simulink library "tqd"  (R2021b)
settings: Solver=VariableStepAuto  StartTime=0.0  StopTime=10.0  RelTol=1e-3
undefined symbols (not defined in the file or in its folder): ATQD_AccelLimitInRange_X_rpm, ATQD_AccelLimitInRange_Y_Nm, ATQD_AccelLimitOvrKi_X_Nm, ATQD_AccelLimitOvrKp_X_Nm, ATQD_BOSMapD_X_rpm, ATQD_BOSMapD_Y_pct, ATQD_BOSMapR_X_rpm, ATQD_BOSMapR_Y_pct, ATQD_HVBCurrSmooth_X_A, ATQD_LHMTqMapDLC_X_rpm, ATQD_LHMTqMapDLC_Y_pct, ATQD_LHMTqMapRLC_X_rpm, ATQD_LHMTqMapRLC_Y_pct, ATQD_NormalMapDLC_X_rpm, ATQD_NormalMapDLC_Y_pct, ATQD_NormalTqDecSR_X_rpm, ATQD_NormalTqDecSR_Y_Nm, ATQD_NormalTqIncSR_X_rpm, ATQD_NormalTqIncSR_Y_Nm, ATQD_OPDMapRLC_X_rpm, ATQD_OPDMapRLC_Y_pct, ATQD_RollRegTorReq_X_rpm, ATQD_RollRegTorReq_Y_enum, ATQD_VehSpdLimitInRange_X_rpm, ATQD_VehSpdLimitInRange_Y_Nm, ATQD_VehSpdLimitOvrKi_X_Nm, ATQD_VehSpdLimitOvrKp_X_Nm, EIGHT_INT, ENUM_BRAKEPEDAL_PRESSED, ENUM_BRAKEPEDAL_RELEASED, ENUM_COMBOKEY_DOWN, ENUM_COMBOKEY_M1, ENUM_COMBOKEY_M2, ENUM_COMBOKEY_NONE, ENUM_COMBOKEY_RKNEE, ENUM_COMBOKEY_STOPLV, ENUM_COMBOKEY_UP, ENUM_CP2VKNEEREQ_REQUEST, ENUM_CP2VNLVREQ_LEVEL1, ENUM_CP2VNLVREQ_LEVEL2, ENUM_CP2VNLVREQ_LOWER, ENUM_CP2VNLVREQ_STOPLV, ENUM_CP2VNLVREQ_UPPER, ENUM_CREEPIND_DISABLE, ENUM_CREEPIND_READY, ENUM_CREEPIND_RUNNING, ENUM_CREEPIND_WARNING, ENUM_DRIVELINERELEASE_RELEASE, ENUM_EBSTORQUERWQ_LIMIT, ENUM_EBSTORQUERWQ_TORQUE, ENUM_ECPVCUDRM_CONFORT, ENUM_ECPVCUDRM_ECO, ENUM_ECPVCUDRM_NORMAL, ENUM_ECPVCUDRM_NOTAVAILABLE, ENUM_EMTqModeDrvBrk_Accel, ENUM_EMTqModeDrvBrk_Brake, ENUM_EMTqModeDrvBrk_Coast, ENUM_ETC2ACTDRIVEDIR_BACKWARD, ENUM_ETC2ACTDRIVEDIR_FORWARD, ENUM_ETC2ACTDRIVEDIR_STILL ... (+341)
libraries: simulink x109, hcu_lib x67
(part 8 of 13)

== system tqd/TQD/OutpConvert/Buzzer Request/Parking Protect Flasher ==
  Task_Time_s : Inport
  ON_s : Inport  Port=2
  OFF_s : Inport  Port=3
  Cycle_cnt : Inport  Port=4
  Wait_s : Inport  Port=5
  VSCP_FlasherEn_flg : Inport  Port=6
  Add : Sum  Inputs=+-
  Chart : Stateflow chart  TreatAsAtomicUnit=on
  Constant4 : Constant  Value=ONE_INT
  Data Type Conversion{,1..3} (4 alike) : DataTypeConversion  OutDataTypeStr=uint8
  Divide : Product  Inputs=*/
  Divide1 : Product  Inputs=*/
  Divide2 : Product  Inputs=*/
  Floor : Rounding
  Floor1 : Rounding
  Floor2 : Rounding
  SigOut : Outport
  wires:
  Floor/1 -> Data Type Conversion/1  "ON_cnt"
  [TaskTime_s] -> Divide2/2
  [Cycle_cnt] -> Add/1  "Cycle_cnt"
  VSCP_FlasherEn_flg/1 -> [VSCP_FlasherEn_flg]
  [VSCP_FlasherEn_flg] -> Chart/5(VSCP_FlasherEn_flg)
  Wait_s/1 -> [Wait_s]
  Task_Time_s/1 -> [TaskTime_s]
  OFF_s/1 -> [OFF_s]
  Cycle_cnt/1 -> [Cycle_cnt]
  [TaskTime_s] -> Divide/2
  [Wait_s] -> Divide2/1  "Wait_s"
  [OFF_s] -> Divide1/1  "OFF_s"
  Constant4/1 -> Add/2
  Data Type Conversion3/1 -> Chart/4(Cycle_cnt)
  ON_s/1 -> [ON_s]
  Divide1/1 -> Floor1/1
  Floor2/1 -> Data Type Conversion2/1  "WAIT_cnt"
  [ON_s] -> Divide/1  "ON_s"
  Data Type Conversion/1 -> Chart/1(ON_cnt)
  Chart/1(out) -> SigOut/1
  Data Type Conversion1/1 -> Chart/2(OFF_cnt)
  Data Type Conversion2/1 -> Chart/3(WAIT_cnt)
  Floor1/1 -> Data Type Conversion1/1  "OFF_cnt"
  Add/1 -> Data Type Conversion3/1  "Cycle_cnt"
  Divide/1 -> Floor/1
  [TaskTime_s] -> Divide1/2
  Divide2/1 -> Floor2/1

== system tqd/TQD/OutpConvert/Buzzer Request/Power Up Fail Flasher ==
  Task_Time_s : Inport
  ON_s : Inport  Port=2
  OFF_s : Inport  Port=3
  Cycle_cnt : Inport  Port=4
  Wait_s : Inport  Port=5
  VSCP_FlasherEn_flg : Inport  Port=6
  Add : Sum  Inputs=+-
  Chart : Stateflow chart  TreatAsAtomicUnit=on
  Constant4 : Constant  Value=ONE_INT
  Data Type Conversion{,1..3} (4 alike) : DataTypeConversion  OutDataTypeStr=uint8
  Divide : Product  Inputs=*/
  Divide1 : Product  Inputs=*/
  Divide2 : Product  Inputs=*/
  Floor : Rounding
  Floor1 : Rounding
  Floor2 : Rounding
  SigOut : Outport
  wires:
  Floor/1 -> Data Type Conversion/1  "ON_cnt"
  [TaskTime_s] -> Divide2/2
  [Cycle_cnt] -> Add/1  "Cycle_cnt"
  VSCP_FlasherEn_flg/1 -> [VSCP_FlasherEn_flg]
  [VSCP_FlasherEn_flg] -> Chart/5(VSCP_FlasherEn_flg)
  Wait_s/1 -> [Wait_s]
  Task_Time_s/1 -> [TaskTime_s]
  OFF_s/1 -> [OFF_s]
  Cycle_cnt/1 -> [Cycle_cnt]
  [TaskTime_s] -> Divide/2
  [Wait_s] -> Divide2/1  "Wait_s"
  [OFF_s] -> Divide1/1  "OFF_s"
  Constant4/1 -> Add/2
  Data Type Conversion3/1 -> Chart/4(Cycle_cnt)
  ON_s/1 -> [ON_s]
  Divide1/1 -> Floor1/1
  Floor2/1 -> Data Type Conversion2/1  "WAIT_cnt"
  [ON_s] -> Divide/1  "ON_s"
  Data Type Conversion/1 -> Chart/1(ON_cnt)
  Chart/1(out) -> SigOut/1
  Data Type Conversion1/1 -> Chart/2(OFF_cnt)
  Data Type Conversion2/1 -> Chart/3(WAIT_cnt)
  Floor1/1 -> Data Type Conversion1/1  "OFF_cnt"
  Add/1 -> Data Type Conversion3/1  "Cycle_cnt"
  Divide/1 -> Floor/1
  [TaskTime_s] -> Divide1/2
  Divide2/1 -> Floor2/1

== system tqd/TQD/OutpConvert/Buzzer Request/Power Up Finished Flasher ==
  Task_Time_s : Inport
  ON_s : Inport  Port=2
  OFF_s : Inport  Port=3
  Cycle_cnt : Inport  Port=4
  Wait_s : Inport  Port=5
  VSCP_FlasherEn_flg : Inport  Port=6
  Add : Sum  Inputs=+-
  Chart : Stateflow chart  TreatAsAtomicUnit=on
  Constant4 : Constant  Value=ONE_INT
  Data Type Conversion{,1..3} (4 alike) : DataTypeConversion  OutDataTypeStr=uint8
  Divide : Product  Inputs=*/
  Divide1 : Product  Inputs=*/
  Divide2 : Product  Inputs=*/
  Floor : Rounding
  Floor1 : Rounding
  Floor2 : Rounding
  SigOut : Outport
  wires:
  Floor/1 -> Data Type Conversion/1  "ON_cnt"
  [TaskTime_s] -> Divide2/2
  [Cycle_cnt] -> Add/1  "Cycle_cnt"
  VSCP_FlasherEn_flg/1 -> [VSCP_FlasherEn_flg]
  [VSCP_FlasherEn_flg] -> Chart/5(VSCP_FlasherEn_flg)
  Wait_s/1 -> [Wait_s]
  Task_Time_s/1 -> [TaskTime_s]
  OFF_s/1 -> [OFF_s]
  Cycle_cnt/1 -> [Cycle_cnt]
  [TaskTime_s] -> Divide/2
  [Wait_s] -> Divide2/1  "Wait_s"
  [OFF_s] -> Divide1/1  "OFF_s"
  Constant4/1 -> Add/2
  Data Type Conversion3/1 -> Chart/4(Cycle_cnt)
  ON_s/1 -> [ON_s]
  Divide1/1 -> Floor1/1
  Floor2/1 -> Data Type Conversion2/1  "WAIT_cnt"
  [ON_s] -> Divide/1  "ON_s"
  Data Type Conversion/1 -> Chart/1(ON_cnt)
  Chart/1(out) -> SigOut/1
  Data Type Conversion1/1 -> Chart/2(OFF_cnt)
  Data Type Conversion2/1 -> Chart/3(WAIT_cnt)
  Floor1/1 -> Data Type Conversion1/1  "OFF_cnt"
  Add/1 -> Data Type Conversion3/1  "Cycle_cnt"
  Divide/1 -> Floor/1
  [TaskTime_s] -> Divide1/2
  Divide2/1 -> Floor2/1

== system tqd/TQD/OutpConvert/Buzzer Request/Power Up Start Flasher ==
  Task_Time_s : Inport
  ON_s : Inport  Port=2
  OFF_s : Inport  Port=3
  Cycle_cnt : Inport  Port=4
  Wait_s : Inport  Port=5
  VSCP_FlasherEn_flg : Inport  Port=6
  Add : Sum  Inputs=+-
  Chart : Stateflow chart  TreatAsAtomicUnit=on
  Constant4 : Constant  Value=ONE_INT
  Data Type Conversion{,1..3} (4 alike) : DataTypeConversion  OutDataTypeStr=uint8
  Divide : Product  Inputs=*/
  Divide1 : Product  Inputs=*/
  Divide2 : Product  Inputs=*/
  Floor : Rounding
  Floor1 : Rounding
  Floor2 : Rounding
  SigOut : Outport
  wires:
  Floor/1 -> Data Type Conversion/1  "ON_cnt"
  [TaskTime_s] -> Divide2/2
  [Cycle_cnt] -> Add/1  "Cycle_cnt"
  VSCP_FlasherEn_flg/1 -> [VSCP_FlasherEn_flg]
  [VSCP_FlasherEn_flg] -> Chart/5(VSCP_FlasherEn_flg)
  Wait_s/1 -> [Wait_s]
  Task_Time_s/1 -> [TaskTime_s]
  OFF_s/1 -> [OFF_s]
  Cycle_cnt/1 -> [Cycle_cnt]
  [TaskTime_s] -> Divide/2
  [Wait_s] -> Divide2/1  "Wait_s"
  [OFF_s] -> Divide1/1  "OFF_s"
  Constant4/1 -> Add/2
  Data Type Conversion3/1 -> Chart/4(Cycle_cnt)
  ON_s/1 -> [ON_s]
  Divide1/1 -> Floor1/1
  Floor2/1 -> Data Type Conversion2/1  "WAIT_cnt"
  [ON_s] -> Divide/1  "ON_s"
  Data Type Conversion/1 -> Chart/1(ON_cnt)
  Chart/1(out) -> SigOut/1
  Data Type Conversion1/1 -> Chart/2(OFF_cnt)
  Data Type Conversion2/1 -> Chart/3(WAIT_cnt)
  Floor1/1 -> Data Type Conversion1/1  "OFF_cnt"
  Add/1 -> Data Type Conversion3/1  "Cycle_cnt"
  Divide/1 -> Floor/1
  [TaskTime_s] -> Divide1/2
  Divide2/1 -> Floor2/1

== system tqd/TQD/Input_Convert/Function/Acceleration Limiter/Limit Torque Calaulation ==
  Refference : Inport
  VehAccel : Inport  Port=2
  PIControl_Task_time : Inport  Port=3
  VTQD_VehAccelTorLimitLast_Nm : Inport  Port=4
  Trigger : TriggerPort  VariantControl=Variant  PortDimensions=1
  Add : Sum
  Add1 : Sum
  Add12 : Sum  Inputs=+-
  MTQD_AccelLimitOvrKi_Y_Gain : Lookup_n-D  NumberOfTableDimensions=1  BreakpointsForDimension1=ATQD_AccelLimitOvrKi_X_Nm  Table=MTQD_AccelLimitOvrKi_Y_Gain  InternalRulePriority=Speed  RndMeth=Simplest  InputSameDT=on
  MTQD_AccelLimitOvrKp_Y_Gain : Lookup_n-D  NumberOfTableDimensions=1  BreakpointsForDimension1=ATQD_AccelLimitOvrKp_X_Nm  Table=MTQD_AccelLimitOvrKp_Y_Gain  InternalRulePriority=Speed  RndMeth=Simplest  InputSameDT=on
  Product : Product
  Product1 : Product
  Product4 : Product
  Sum8 : Sum
  Unit Delay13 : UnitDelay  InitialCondition=single(0)  SampleTime=-1  HasFrameUpgradeWarning=on
      settings: AttributesFormatString=%<InitialCondition>
  Result : Outport
  wires:
  Product4/1 -> Sum8/2
  Product/1 -> Add1/1, Product1/1
  Sum8/1 -> Unit Delay13/1, Add1/2
  Add12/1 -> Product/1  "error"
  Unit Delay13/1 -> Sum8/1
  Product1/1 -> Product4/1
  Refference/1 -> Add12/1
  VehAccel/1 -> Add12/2
  PIControl_Task_time/1 -> Product4/2
  VTQD_VehAccelTorLimitLast_Nm/1 -> [VTQD_VehAccelTorLimitLast_Nm]
  [VTQD_VehAccelTorLimitLast_Nm] -> MTQD_AccelLimitOvrKi_Y_Gain/1, MTQD_AccelLimitOvrKp_Y_Gain/1
  MTQD_AccelLimitOvrKp_Y_Gain/1 -> [VTQD_VehAccelLimitOvrKp_Gain]  "VTQD_AccelLimitOvrKp_Gain"
  MTQD_AccelLimitOvrKi_Y_Gain/1 -> [VTQD_VehAccelLimitOvrKi_Gain]  "VTQD_AceelLimitOvrKi_Gain"
  [VTQD_VehAccelLimitOvrKp_Gain] -> Product/2
  [VTQD_VehAccelLimitOvrKi_Gain] -> Product1/2
  [VTQD_VehAccelTorLimitLast_Nm] -> Add/1
  Add1/1 -> Add/2
  Add/1 -> Result/1

== system tqd/TQD/Input_Convert/Function/Acceleration Limiter/Vehicle Acceleration Calculation ==
  VTQD_VCUVehSpd_kph : Inport
  VTQD_tasktime_s : Inport  Port=2
  KTQD_VehAccelCalDeltaT_s : Inport  Port=3
  KTQD_VehAccelCalFilterTs_s : Inport  Port=4
  Trigger : TriggerPort  VariantControl=Variant  PortDimensions=1
  Add1 : Sum  Inputs=+-
  Constant13 : Constant  Value=EPS
  Divide1 : Product  Inputs=*/
  FirstOrderFilter1 : hcu_lib/Basic_Blocks/FirstOrderFilter
      settings: SourceProductName=HCU Relative Block Library
  KPH2MPS : Gain  Gain=KPH2MPS  OutDataTypeStr=single
  Max : MinMax  Function=max  Inputs=2
  Unit Delay1 : UnitDelay  InitialCondition=single(0)  SampleTime=-1  HasFrameUpgradeWarning=on
      settings: AttributesFormatString=%<InitialCondition>
  VTQD_VehAccel_mps2 : Outport
  wires:
  Unit Delay1/1 -> Add1/2
  VTQD_tasktime_s/1 -> FirstOrderFilter1/2
  KTQD_VehAccelCalFilterTs_s/1 -> FirstOrderFilter1/3
  FirstOrderFilter1/1 -> VTQD_VehAccel_mps2/1
  Divide1/1 -> FirstOrderFilter1/1
  VTQD_VCUVehSpd_kph/1 -> Unit Delay1/1, Add1/1
  Max/1 -> Divide1/2
  KTQD_VehAccelCalDeltaT_s/1 -> Max/1
  Constant13/1 -> Max/2
  Add1/1 -> KPH2MPS/1
  KPH2MPS/1 -> Divide1/1

== system tqd/TQD/Input_Convert/Function/Speed Limiter/Limit Torque Calculation ==
  Refference : Inport
  VDIP_VCUVehSpd_kph : Inport  Port=2
  PIControl_Task_time : Inport  Port=3
  VTQD_VehSpdTorLimitLast_Nm : Inport  Port=4
  Trigger : TriggerPort  VariantControl=Variant  PortDimensions=1
  Add : Sum
  Add12 : Sum  Inputs=+-
  MTQD_VehSpdLimitOvrKi_Y_Gain : Lookup_n-D  NumberOfTableDimensions=1  BreakpointsForDimension1=ATQD_VehSpdLimitOvrKi_X_Nm  Table=MTQD_VehSpdLimitOvrKi_Y_Gain  InternalRulePriority=Speed  RndMeth=Simplest  InputSameDT=on
  MTQD_VehSpdLimitOvrKp_Y_Gain : Lookup_n-D  NumberOfTableDimensions=1  BreakpointsForDimension1=ATQD_VehSpdLimitOvrKp_X_Nm  Table=MTQD_VehSpdLimitOvrKp_Y_Gain  InternalRulePriority=Speed  RndMeth=Simplest  InputSameDT=on
  Product : Product
  Product1 : Product
  Product4 : Product
  Sum6 : Sum
  Sum8 : Sum
  Unit Delay13 : UnitDelay  InitialCondition=single(0)  SampleTime=-1  HasFrameUpgradeWarning=on
      settings: AttributesFormatString=%<InitialCondition>
  Result : Outport
  wires:
  Product4/1 -> Sum8/2
  Product/1 -> Product1/1, Sum6/1
  Sum8/1 -> Unit Delay13/1, Sum6/2
  Add12/1 -> Product/1  "error"
  Unit Delay13/1 -> Sum8/1
  Product1/1 -> Product4/1
  Refference/1 -> Add12/1
  VDIP_VCUVehSpd_kph/1 -> Add12/2
  PIControl_Task_time/1 -> Product4/2
  VTQD_VehSpdTorLimitLast_Nm/1 -> [VTQD_VehSpdTorLimitLast_Nm]
  [VTQD_VehSpdTorLimitLast_Nm] -> MTQD_VehSpdLimitOvrKi_Y_Gain/1, MTQD_VehSpdLimitOvrKp_Y_Gain/1
  MTQD_VehSpdLimitOvrKp_Y_Gain/1 -> [VTQD_VehSpdLimitOvrKp_Gain]  "VTQD_VehSpdLimitOvrKp_Gain"
  MTQD_VehSpdLimitOvrKi_Y_Gain/1 -> [VTQD_VehSpdLimitOvrKi_Gain]  "VTQD_VehSpdLimitOvrKi_Gain"
  [VTQD_VehSpdLimitOvrKp_Gain] -> Product/2
  [VTQD_VehSpdLimitOvrKi_Gain] -> Product1/2
  [VTQD_VehSpdTorLimitLast_Nm] -> Add/1
  Sum6/1 -> Add/2
  Add/1 -> Result/1

== system tqd/TQD/Input_Convert/Input Signal Convert/Big Mike Combo V2 /Combo Key Detection ==
  task_time_s : Inport
  VTQD_ComboKeyEn_flg : Inport  Port=2
  VTQD_ComboKeyReset_flg : Inport  Port=3
  VTQD_ComboKey_enum : Inport  Port=4
  VTQD_ComboKeyEnter_flg : Inport  Port=5
  VTQD_ComboKeyOff_flg : Inport  Port=6
  Function1 Alcohol Lock : Subsystem
      settings: RTWSystemCode=Nonreusable function
  "Function2 " : Subsystem
      settings: RTWSystemCode=Nonreusable function
  Function3 : Subsystem
      settings: RTWSystemCode=Nonreusable function
  "Function4 " : Subsystem
      settings: RTWSystemCode=Nonreusable function
  Function5 : Subsystem
      settings: RTWSystemCode=Nonreusable function
  VTQD_Function1Off_flg : Outport
  VTQD_Function2Off_flg : Outport  Port=2
  VTQD_Function3Off_flg : Outport  Port=3
  VTQD_Function4Off_flg : Outport  Port=4
  VTQD_Function5Off_flg : Outport  Port=5
  wires:
  [VTQD_ComboKeyEn_flg] -> Function1 Alcohol Lock/2(VTQD_ComboKeyEn_flg)
  [VTQD_ComboKeyOff_flg] -> Function1 Alcohol Lock/6(VTQD_ComboKeyOff_flg)
  Function1 Alcohol Lock/1(VTQD_Function1Off_flg) -> [VTQD_Function1Off_flg]
  [VTQD_ComboKeyReset_flg] -> Function1 Alcohol Lock/3(VTQD_ComboKeyReset_flg)
  [task_time_s] -> Function1 Alcohol Lock/1(task_time_s)
  [VTQD_ComboKeyEnter_flg] -> Function1 Alcohol Lock/5(VTQD_ComboKeyEnter_flg)
  [VTQD_ComboKey_enum] -> Function1 Alcohol Lock/4(VTQD_ComboKey_enum)
  task_time_s/1 -> [task_time_s]
  VTQD_ComboKeyEn_flg/1 -> [VTQD_ComboKeyEn_flg]
  VTQD_ComboKeyReset_flg/1 -> [VTQD_ComboKeyReset_flg]
  VTQD_ComboKey_enum/1 -> [VTQD_ComboKey_enum]
  VTQD_ComboKeyEnter_flg/1 -> [VTQD_ComboKeyEnter_flg]
  VTQD_ComboKeyOff_flg/1 -> [VTQD_ComboKeyOff_flg]
  [VTQD_ComboKey_enum] -> "Function2 "/4(VTQD_ComboKey_enum)
  [VTQD_ComboKeyEnter_flg] -> "Function2 "/5(VTQD_ComboKeyEnter_flg)
  [task_time_s] -> "Function2 "/1(task_time_s)
  [VTQD_ComboKeyReset_flg] -> "Function2 "/3(VTQD_ComboKeyReset_flg)
  "Function2 "/1(VTQD_Function2Off_flg) -> [VTQD_Function2Off_flg]
  [VTQD_ComboKeyOff_flg] -> "Function2 "/6(VTQD_ComboKeyOff_flg)
  [VTQD_ComboKeyEn_flg] -> "Function2 "/2(VTQD_ComboKeyEn_flg)
  [VTQD_Function1Off_flg] -> VTQD_Function1Off_flg/1
  [VTQD_Function2Off_flg] -> VTQD_Function2Off_flg/1
  [VTQD_ComboKeyEn_flg] -> Function3/2(VTQD_ComboKeyEn_flg)
  [VTQD_ComboKeyOff_flg] -> Function3/6(VTQD_ComboKeyOff_flg)
  [VTQD_ComboKeyReset_flg] -> Function3/3(VTQD_ComboKeyReset_flg)
  [task_time_s] -> Function3/1(task_time_s)
  [VTQD_ComboKeyEnter_flg] -> Function3/5(VTQD_ComboKeyEnter_flg)
  [VTQD_ComboKey_enum] -> Function3/4(VTQD_ComboKey_enum)
  Function3/1(VTQD_Function3Off_flg) -> [VTQD_Function3Off_flg]
  [VTQD_ComboKey_enum] -> "Function4 "/4(VTQD_ComboKey_enum)
  [VTQD_ComboKeyEnter_flg] -> "Function4 "/5(VTQD_ComboKeyEnter_flg)
  [task_time_s] -> "Function4 "/1(task_time_s)
  [VTQD_ComboKeyReset_flg] -> "Function4 "/3(VTQD_ComboKeyReset_flg)
  [VTQD_ComboKeyOff_flg] -> "Function4 "/6(VTQD_ComboKeyOff_flg)
  [VTQD_ComboKeyEn_flg] -> "Function4 "/2(VTQD_ComboKeyEn_flg)
  "Function4 "/1(VTQD_Function4Off_flg) -> [VTQD_Function4Off_flg]
  [VTQD_Function3Off_flg] -> VTQD_Function3Off_flg/1
  [VTQD_Function4Off_flg] -> VTQD_Function4Off_flg/1
  [VTQD_ComboKeyEn_flg] -> Function5/2(VTQD_ComboKeyEn_flg)
  [VTQD_ComboKeyOff_flg] -> Function5/6(VTQD_ComboKeyOff_flg)
  [VTQD_ComboKeyReset_flg] -> Function5/3(VTQD_ComboKeyReset_flg)
  [task_time_s] -> Function5/1(task_time_s)
  [VTQD_ComboKeyEnter_flg] -> Function5/5(VTQD_ComboKeyEnter_flg)
  [VTQD_ComboKey_enum] -> Function5/4(VTQD_ComboKey_enum)
  Function5/1(VTQD_Function5Off_flg) -> [VTQD_Function5Off_flg]
  [VTQD_Function5Off_flg] -> VTQD_Function5Off_flg/1

== system tqd/TQD/Input_Convert/Input Signal Convert/Big Mike Combo V2 /Mode Coordination ==
  VTQD_Function1Off_flg : Inport
  VTQD_Function2Off_flg : Inport  Port=2
  VTQD_Function3Off_flg : Inport  Port=3
  VTQD_Function4Off_flg : Inport  Port=4
  VTQD_Function5Off_flg : Inport  Port=5
  Add : Sum  Inputs=+++++
  Constant : Constant  Value=ONE_INT
  Constant{1..6} (6 alike) : Constant  Value=ZERO_INT
  Constant7 : Constant  Value=SIXTEEN_INT
  Constant8 : Constant  Value=FOUR_INT
  Constant9 : Constant  Value=EIGHT_INT
  Data Type Conversion : DataTypeConversion  OutDataTypeStr=uint8
  Switch{,1..4} (5 alike) : Switch  Criteria=u2 ~= 0
      settings: AttributesFormatString=%<Criteria>
  VTQD_FunctionOffSta_enum : Outport
  wires:
  VTQD_Function1Off_flg/1 -> [VTQD_Function1Off_flg]
  VTQD_Function2Off_flg/1 -> [VTQD_Function2Off_flg]
  VTQD_Function3Off_flg/1 -> [VTQD_Function3Off_flg]
  VTQD_Function4Off_flg/1 -> [VTQD_Function4Off_flg]
  VTQD_Function5Off_flg/1 -> [VTQD_Function5Off_flg]
  Add/1 -> Data Type Conversion/1
  [VTQD_FunctionOffSta_enum] -> VTQD_FunctionOffSta_enum/1
  [VTQD_Function1Off_flg] -> Switch/2
  Constant/1 -> Switch/1
  Constant1/1 -> Switch/3
  Constant2/1 -> Switch1/3
  Constant6/1 -> Switch1/1
  Constant8/1 -> Switch2/1
  Constant4/1 -> Switch2/3
  Constant3/1 -> Switch3/3
  Constant9/1 -> Switch3/1
  Constant7/1 -> Switch4/1
  Constant5/1 -> Switch4/3
  [VTQD_Function2Off_flg] -> Switch1/2
  [VTQD_Function3Off_flg] -> Switch2/2
  [VTQD_Function4Off_flg] -> Switch3/2
  [VTQD_Function5Off_flg] -> Switch4/2
  Switch2/1 -> Add/3
  Switch1/1 -> Add/2
  Switch/1 -> Add/1
  Switch3/1 -> Add/4
  Switch4/1 -> Add/5
  Data Type Conversion/1 -> [VTQD_FunctionOffSta_enum]  "VTQD_FunctionOffSta_enum"

== system tqd/TQD/Input_Convert/Input Signal Convert/Big Mike Combo V2 /Operation Condition ==
  VPMM_SysPowerMode_enum : Inport
  VTQD_GearActualPosn_enum : Inport  Port=2
  VTQD_ComboKeyEnCMD_flg : Inport  Port=3
  VINP_ParkBrakeSW_flg : Inport  Port=4
  VTQD_ActFRDoorOPSta_flg : Inport  Port=5
  AND : Logic  Inputs=4  AllPortsSameDT=off  OutDataTypeStr=boolean
  AND1 : Logic  AllPortsSameDT=off  OutDataTypeStr=boolean
  Constant1 : Constant  Value=ENUM_PMMMODE_STANDBY
  Constant2 : Constant  Value=ENUM_PMMMODE_STANDBY
  Constant3 : Constant  Value=ENUM_GEARACTUALPOSN_N
  Constant4 : Constant  Value=ENUM_GEARACTUALPOSN_P
  Equal : RelationalOperator  Operator===  OutDataTypeStr=boolean  RndMeth=Simplest
  Equal1 : RelationalOperator  Operator=~=  OutDataTypeStr=boolean  RndMeth=Simplest
  Equal2 : RelationalOperator  Operator===  OutDataTypeStr=boolean  RndMeth=Simplest
  Equal3 : RelationalOperator  Operator===  OutDataTypeStr=boolean  RndMeth=Simplest
  NOT : Logic  Operator=NOT  AllPortsSameDT=off  OutDataTypeStr=boolean
  NOT1 : Logic  Operator=NOT  AllPortsSameDT=off  OutDataTypeStr=boolean
  OR1 : Logic  Operator=OR  AllPortsSameDT=off  OutDataTypeStr=boolean
  OR2 : Logic  Operator=OR  Inputs=3  AllPortsSameDT=off  OutDataTypeStr=boolean
  SR_Latch : hcu_lib/Basic_Blocks/SR_Latch
  VTQD_ComboKeyPreEn_flg : Outport
  VTQD_ComboKeyEn_flg : Outport  Port=2
  wires:
  Equal/1 -> AND/1
  Equal2/1 -> OR1/1
  Constant3/1 -> Equal3/2
  [VTQD_GearActualPosn_enum] -> Equal2/1
  Equal3/1 -> OR1/2
  Constant4/1 -> Equal2/2
  [VTQD_GearActualPosn_enum] -> Equal3/1
  [VPMM_SysPowerMode_enum] -> Equal/1
  Constant2/1 -> Equal/2
  VPMM_SysPowerMode_enum/1 -> [VPMM_SysPowerMode_enum]
  VTQD_GearActualPosn_enum/1 -> [VTQD_GearActualPosn_enum]
  [VTQD_ComboKeyPreEn_flg] -> VTQD_ComboKeyPreEn_flg/1
  VTQD_ComboKeyEnCMD_flg/1 -> [VTQD_ComboKeyEnCMD_flg]
  [VTQD_ComboKeyPreEn_flg] -> AND1/1
  [VTQD_ComboKeyEnCMD_flg] -> AND1/2
  AND1/1 -> [VTQD_ComboKeyEn_flg]  "VTQD_ComboKeyEn_flg"
  [VTQD_ComboKeyEn_flg] -> VTQD_ComboKeyEn_flg/1
  VINP_ParkBrakeSW_flg/1 -> [VINP_ParkBrakeSW_flg]
  VTQD_ActFRDoorOPSta_flg/1 -> [VTQD_ActFRDoorOPSta_flg]
  [VINP_ParkBrakeSW_flg] -> AND/2
  [VTQD_ActFRDoorOPSta_flg] -> AND/3
  OR1/1 -> AND/4
  AND/1 -> SR_Latch/1  "VTQD_ComboKeyPreEnSet_flg"
  SR_Latch/1 -> [VTQD_ComboKeyPreEn_flg]  "VTQD_ComboKeyPreEn_flg"
  Constant1/1 -> Equal1/2
  [VPMM_SysPowerMode_enum] -> Equal1/1
  [VINP_ParkBrakeSW_flg] -> NOT/1
  Equal1/1 -> OR2/1
  NOT/1 -> OR2/2
  OR2/1 -> SR_Latch/2  "VTQD_ComboKeyPreEnReset_flg"
  [VTQD_ActFRDoorOPSta_flg] -> NOT1/1
  NOT1/1 -> OR2/3

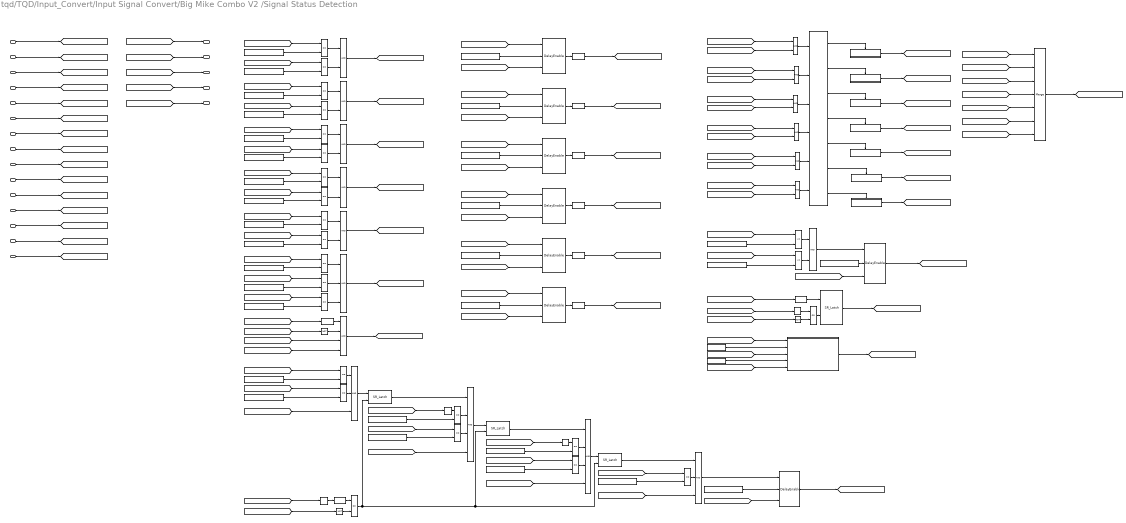
== system tqd/TQD/Input_Convert/Input Signal Convert/Big Mike Combo V2 /Signal Status Detection ==
  note: Combo Key Note:
      | ENUM_COMBOKEY_NONE = uint8(0); None
      | ENUM_COMBOKEY_UP = uint8(1); ECASUp
      | ENUM_COMBOKEY_DOWN = uint8(2); ECASDown
      | ENUM_COMBOKEY_STOPLV = uint8(3); ECASStopLV
      | ENUM_COMBOKEY_M1 = uint8(4); ECASM1
      | ENUM_COMBOKEY_M2 = uint8(5); ECASM2
      | ENUM_COMBOKEY_RKNEE = uint8(6); ECASRKnee
  task_time_s : Inport
  VACC_ASC2NLvReqFA_enum : Inport  Port=2
  VACC_ASC2NLvReqRA_enum : Inport  Port=3
  VACC_ASC2KneeReqRSide_flg : Inport  Port=4
  VACC_ASC2KneeReqFA_flg : Inport  Port=5
  VACC_ASC2KneeReqRA_flg : Inport  Port=6
  VBCM_FDCBCMFDCloseSVCmd_flg : Inport  Port=7
  VBCM_FDCBCMFDOpenSVCmd_flg : Inport  Port=8
  VTQD_ComboKeyPreEn_flg : Inport  Port=9
  VINP_TransReqGear_enum : Inport  Port=10
  VTQD_FunctionOffSta_enum : Inport  Port=11
  VDHP_ActAPSPosn_pct : Inport  Port=12
  VINP_BrakePedalPos_pct : Inport  Port=13
  VTQD_ComboKeyEn_flg : Inport  Port=14
  VTQD_ActFRDoorOPSta_flg : Inport  Port=15
  AND{,1..6,15..19} (12 alike) : Logic  AllPortsSameDT=off  OutDataTypeStr=boolean
  AND10 : Logic  Inputs=4  AllPortsSameDT=off  OutDataTypeStr=boolean
  AND11 : Logic  Inputs=4  AllPortsSameDT=off  OutDataTypeStr=boolean
  AND12 : Logic  Inputs=3  AllPortsSameDT=off  OutDataTypeStr=boolean
  AND20 : Logic  Inputs=3  AllPortsSameDT=off  OutDataTypeStr=boolean
  AND7 : Logic  Inputs=3  AllPortsSameDT=off  OutDataTypeStr=boolean
  AND9 : Logic  Inputs=4  AllPortsSameDT=off  OutDataTypeStr=boolean
  Constant{,1..5} (6 alike) : Constant  Value=KTQD_SetSpdShortPLim_s
  Constant10 : Constant  Value=ENUM_TARGETGEAR_REVERSE
  Constant11 : Constant  Value=ENUM_CP2VNLVREQ_UPPER
  Constant12 : Constant  Value=ENUM_CP2VNLVREQ_UPPER
  Constant13 : Constant  Value=ENUM_CP2VNLVREQ_LOWER
  Constant14 : Constant  Value=ENUM_CP2VNLVREQ_LOWER
  Constant15 : Constant  Value=ENUM_CP2VNLVREQ_STOPLV
  Constant16 : Constant  Value=KTQD_ComboKeyAPSPedEn_pct
  Constant17 : Constant  Value=KTQD_ComboKeyBPSPedEn_pct
  Constant18 : Constant  Value=KTQD_ComboKeyEnDelayTime_s
  Constant19 : Constant  Value=ENUM_CP2VNLVREQ_STOPLV
  Constant20 : Constant  Value=ENUM_CP2VNLVREQ_LEVEL1
  Constant21 : Constant  Value=ENUM_CP2VNLVREQ_LEVEL1
  Constant22 : Constant  Value=ENUM_CP2VNLVREQ_LEVEL2
  Constant23 : Constant  Value=ENUM_CP2VNLVREQ_LEVEL2
  Constant24 : Constant  Value=ENUM_CP2VKNEEREQ_REQUEST
  Constant25 : Constant  Value=ENUM_CP2VKNEEREQ_REQUEST
  Constant26 : Constant  Value=ENUM_CP2VKNEEREQ_REQUEST
  Constant27 : Constant  Value=ENUM_TARGETGEAR_NEUTRAL
  Constant28 : Constant  Value=ENUM_TARGETGEAR_NEUTRAL
  Constant29 : Constant  Value=KTQD_EnterKeyCheckTime_s
  Constant30 : Constant  Value=FALSE
  Constant31 : Constant  Value=FALSE
  Constant6 : Constant  Value=ENUM_TARGETGEAR_NEUTRAL
  Constant7 : Constant  Value=ENUM_TARGETGEAR_DRIVE
  Constant8 : Constant  Value=ENUM_TARGETGEAR_DRIVE
  Constant9 : Constant  Value=ENUM_TARGETGEAR_REVERSE
  Delay : Delay  DelayLength=1  InitialCondition=boolean(0)
      settings: AttributesFormatString=%<InitialCondition>
  Delay2 : Delay  DelayLength=1  InitialCondition=uint8(0)
      settings: AttributesFormatString=%<InitialCondition>
  Delay3 : Delay  DelayLength=1  InitialCondition=uint8(0)
      settings: AttributesFormatString=%<InitialCondition>
  Delay4 : Delay  DelayLength=1  InitialCondition=boolean(0)
      settings: AttributesFormatString=%<InitialCondition>
  DelayEnable{,1..6,16} (8 alike) : hcu_lib/Basic_Blocks/DelayEnable
  Detect Decrease{,1..6} (7 alike) : simulink/Logic and Bit Operations/Detect Decrease  vinit=boolean(0)  OutDataTypeStr=boolean
  Detect Increase : simulink/Logic and Bit Operations/Detect Increase  vinit=boolean(0)  OutDataTypeStr=boolean
  Detect Increase1 : simulink/Logic and Bit Operations/Detect Increase  vinit=boolean(0)  OutDataTypeStr=boolean
  DownShort : Subsystem  TreatAsAtomicUnit=on
  Equal{,1..19} (20 alike) : RelationalOperator  Operator===  OutDataTypeStr=boolean  RndMeth=Simplest
  If : If  NumInputs=6  IfExpression=u1~=0  ElseIfExpressions=u2~=0,u3~=0,u4~=0,u5~=0,u6~=0
  M1Short : Subsystem  TreatAsAtomicUnit=on
  M2Short : Subsystem  TreatAsAtomicUnit=on
  Merge : Merge  Inputs=7
  NOT : Logic  Operator=NOT  AllPortsSameDT=off  OutDataTypeStr=boolean
  NOT1 : Logic  Operator=NOT  AllPortsSameDT=off  OutDataTypeStr=boolean
  NOT2 : Logic  Operator=NOT  AllPortsSameDT=off  OutDataTypeStr=boolean
  None : Subsystem  TreatAsAtomicUnit=on
  OR : Logic  Operator=OR  AllPortsSameDT=off  OutDataTypeStr=boolean
  OR1 : Logic  Operator=OR  AllPortsSameDT=off  OutDataTypeStr=boolean
  RKneeShort : Subsystem  TreatAsAtomicUnit=on
  Relational Operator : RelationalOperator  OutDataTypeStr=boolean  RndMeth=Simplest
  Relational Operator1 : RelationalOperator  OutDataTypeStr=boolean  RndMeth=Simplest
  SR_Latch{,1..3} (4 alike) : hcu_lib/Basic_Blocks/SR_Latch
  StopLVShort : Subsystem  TreatAsAtomicUnit=on
  Street Fight Switch Off : Subsystem
      settings: RTWSystemCode=Nonreusable function
  UpShort : Subsystem  TreatAsAtomicUnit=on
  VTQD_ComboKey_enum : Outport
  VTQD_ComboKeyEnCMD_flg : Outport  Port=2
  VTQD_ComboKeyReset_flg : Outport  Port=3
  VTQD_ComboKeyEnter_flg : Outport  Port=4
  VTQD_ComboKeyOff_flg : Outport  Port=5
  wires:
  [VTQD_ComboKey_enum] -> VTQD_ComboKey_enum/1
  Constant/1 -> DelayEnable/2
  DownShort/1(DownShort) -> [DownShort]  "DownShort"
  [M2Short] -> Merge/5
  VACC_ASC2KneeReqRSide_flg/1 -> [VACC_ASC2KneeReqRSide_flg]
  M2Short/1(M2Short) -> [M2Short]  "M2Short"
  Detect Decrease3/1 -> [VTQD_M1Short_flg]  "VTQD_M1Short_flg"
  Detect Decrease5/1 -> [VTQD_RKneeShort_flg]  "VTQD_RKneeShort_flg"
  If/2 -> DownShort/Action
  Constant2/1 -> DelayEnable2/2
  DelayEnable4/1 -> Detect Decrease4/1
  Detect Decrease4/1 -> [VTQD_M2Short_flg]  "VTQD_M2Short_flg"
  DelayEnable5/1 -> Detect Decrease5/1
  Constant5/1 -> DelayEnable5/2
  If/6 -> RKneeShort/Action
  [task_time_s] -> DelayEnable3/3
  [M1Short] -> Merge/4
  [task_time_s] -> DelayEnable5/3
  Constant3/1 -> DelayEnable3/2
  VACC_ASC2NLvReqFA_enum/1 -> [VACC_ASC2NLvReqFA_enum]
  [STOPLV] -> Merge/3
  DelayEnable3/1 -> Detect Decrease3/1
  If/5 -> M2Short/Action
  Detect Decrease/1 -> [VTQD_UpShort_flg]  "VTQD_UpShort_flg"
  task_time_s/1 -> [task_time_s]
  [task_time_s] -> DelayEnable4/3
  If/7 -> None/Action
  Detect Decrease2/1 -> [VTQD_StopLVShort_flg]  "VTQD_StopLVShort_flg"
  If/4 -> M1Short/Action
  Detect Decrease1/1 -> [VTQD_DownShort_flg]  "VTQD_DownShort_flg"
  VBCM_FDCBCMFDCloseSVCmd_flg/1 -> [VBCM_FDCBCMFDCloseSVCmd_flg]
  Constant4/1 -> DelayEnable4/2
  [DownShort] -> Merge/2
  If/1 -> UpShort/Action
  Constant1/1 -> DelayEnable1/2
  [task_time_s] -> DelayEnable/3
  VACC_ASC2KneeReqFA_flg/1 -> [VACC_ASC2KneeReqFA_flg]
  [RKneeShort] -> Merge/6
  VACC_ASC2NLvReqRA_enum/1 -> [VACC_ASC2NLvReqRA_enum]
  DelayEnable/1 -> Detect Decrease/1
  [task_time_s] -> DelayEnable2/3
  DelayEnable2/1 -> Detect Decrease2/1
  VACC_ASC2KneeReqRA_flg/1 -> [VACC_ASC2KneeReqRA_flg]
  [UpShort] -> Merge/1
  None/1(None) -> [None]  "None"
  [task_time_s] -> DelayEnable1/3
  DelayEnable1/1 -> Detect Decrease1/1
  If/3 -> StopLVShort/Action
  UpShort/1(UpShort) -> [UpShort]  "UpShort"
  StopLVShort/1(STOPLV) -> [STOPLV]  "StopLVShort"
  M1Short/1(M1Short) -> [M1Short]  "M1Short"
  Merge/1 -> [VTQD_ComboKey_enum]  "VTQD_ComboKey_enum"
  RKneeShort/1(RKneeShort) -> [RKneeShort]  "RKneeShort"
  SR_Latch/1 -> [VTQD_ComboKeyEnCMD_flg]  "VTQD_ComboKeyEnCMD_flg"
  VBCM_FDCBCMFDOpenSVCmd_flg/1 -> [VBCM_FDCBCMFDOpenSVCmd_flg]
  [VTQD_ComboKeyEnCMD_flg] -> VTQD_ComboKeyEnCMD_flg/1
  VTQD_ComboKeyPreEn_flg/1 -> [VTQD_ComboKeyPreEn_flg]
  AND1/1 -> If/1
  [VTQD_ComboKeyPreEn_flg] -> AND1/2
  AND2/1 -> If/2
  [VTQD_ComboKeyPreEn_flg] -> AND2/2
  AND3/1 -> If/3
  [VTQD_StopLVShort_flg] -> AND3/1
  [VTQD_ComboKeyPreEn_flg] -> AND3/2
  AND4/1 -> If/4
  [VTQD_ComboKeyPreEn_flg] -> AND4/2
  AND5/1 -> If/5
  [VTQD_ComboKeyPreEn_flg] -> AND5/2
  AND6/1 -> If/6
  [VTQD_ComboKeyPreEn_flg] -> AND6/2
  VINP_TransReqGear_enum/1 -> [VINP_TransReqGear_enum]
  [VTQD_ComboKeyReset_flg] -> VTQD_ComboKeyReset_flg/1
  [VTQD_ComboKeyEnter_flg] -> VTQD_ComboKeyEnter_flg/1
  DelayEnable6/1 -> [VTQD_ComboKeyEnter_flg]  "VTQD_ComboKeyEnter_flg"
  Street Fight Switch Off/1(VTQD_ComboKeyOff_flg) -> [VTQD_ComboKeyOff_flg]
  [task_time_s] -> Street Fight Switch Off/1(task_time_s)
  [VTQD_ComboKeyPreEn_flg] -> Street Fight Switch Off/3(VTQD_ComboKeyPreEn_flg)
  [VTQD_ComboKeyOff_flg] -> VTQD_ComboKeyOff_flg/1
  VTQD_FunctionOffSta_enum/1 -> [VTQD_FunctionOffSta_enum]
  [VTQD_FunctionOffSta_enum] -> Street Fight Switch Off/5(VTQD_FunctionOffSta_enum)
  VDHP_ActAPSPosn_pct/1 -> [VDHP_ActAPSPosn_pct]
  VINP_BrakePedalPos_pct/1 -> [VINP_BrakePedalPos_pct]
  [None] -> Merge/7
  [VTQD_UpShort_flg] -> AND1/1
  [VTQD_M1Short_flg] -> AND4/1
  [VTQD_M2Short_flg] -> AND5/1
  [VTQD_RKneeShort_flg] -> AND6/1
  VTQD_ComboKeyEn_flg/1 -> [VTQD_ComboKeyEn_flg]
  [VDHP_ActAPSPosn_pct] -> Relational Operator/1
  Constant16/1 -> Relational Operator/2
  Constant17/1 -> Relational Operator1/2
  [VINP_BrakePedalPos_pct] -> Relational Operator1/1
  Relational Operator/1 -> AND/1
  Relational Operator1/1 -> AND/2
  AND/1 -> DelayEnable16/1
  [task_time_s] -> DelayEnable16/3
  Constant18/1 -> DelayEnable16/2
  NOT/1 -> OR/2
  [VTQD_ComboKeyPreEn_flg] -> NOT/1
  DelayEnable16/1 -> [VTQD_ComboKeyEnCMDSta_flg]  "VTQD_ComboKeyEnCMDSta_flg"
  [VTQD_ComboKeyEnCMDSta_flg] -> Detect Increase/1
  Detect Increase/1 -> SR_Latch/1
  OR/1 -> SR_Latch/2
  [VACC_ASC2NLvReqFA_enum] -> Equal/1
  [VACC_ASC2NLvReqRA_enum] -> Equal1/1
  Constant12/1 -> Equal1/2
  Constant11/1 -> Equal/2
  Equal/1 -> AND15/1
  Equal1/1 -> AND15/2
  AND15/1 -> [VTQD_ECPECASUp_flg]  "VTQD_ECPECASUp_flg"
  [VTQD_ECPECASUp_flg] -> DelayEnable/1
  AND16/1 -> [VTQD_ECPECASDown_flg]  "VTQD_ECPECASDown_flg"
  Equal3/1 -> AND16/2
  Equal2/1 -> AND16/1
  Constant13/1 -> Equal2/2
  Constant14/1 -> Equal3/2
  [VACC_ASC2NLvReqRA_enum] -> Equal3/1
  [VACC_ASC2NLvReqFA_enum] -> Equal2/1
  [VACC_ASC2NLvReqFA_enum] -> Equal4/1
  [VACC_ASC2NLvReqRA_enum] -> Equal5/1
  Constant19/1 -> Equal5/2
  Constant15/1 -> Equal4/2
  Equal4/1 -> AND17/1
  Equal5/1 -> AND17/2
  AND17/1 -> [VTQD_ECPECASStopLV_flg]  "VTQD_ECPECASStopLV_flg"
  AND18/1 -> [VTQD_ECPECASM1_flg]  "VTQD_ECPECASM1_flg"
  Equal7/1 -> AND18/2
  Equal6/1 -> AND18/1
  Constant20/1 -> Equal6/2
  Constant21/1 -> Equal7/2
  [VACC_ASC2NLvReqRA_enum] -> Equal7/1
  [VACC_ASC2NLvReqFA_enum] -> Equal6/1
  [VACC_ASC2NLvReqFA_enum] -> Equal8/1
  [VACC_ASC2NLvReqRA_enum] -> Equal9/1
  Constant23/1 -> Equal9/2
  Constant22/1 -> Equal8/2
  Equal8/1 -> AND19/1
  Equal9/1 -> AND19/2
  AND19/1 -> [VTQD_ECPECASM2_flg]  "VTQD_ECPECASM2_flg"
  [VTQD_ECPECASDown_flg] -> DelayEnable1/1
  [VTQD_DownShort_flg] -> AND2/1
  [VTQD_ECPECASStopLV_flg] -> DelayEnable2/1
  [VTQD_ECPECASM1_flg] -> DelayEnable3/1
  [VTQD_ECPECASM2_flg] -> DelayEnable4/1
  Equal11/1 -> AND20/2
  Equal10/1 -> AND20/1
  Constant24/1 -> Equal10/2
  Constant25/1 -> Equal11/2
  [VACC_ASC2KneeReqFA_flg] -> Equal11/1
  [VACC_ASC2KneeReqRSide_flg] -> Equal10/1
  [VACC_ASC2KneeReqRA_flg] -> Equal12/1
  Constant26/1 -> Equal12/2
  Equal12/1 -> AND20/3
  AND20/1 -> [VTQD_ECPECASRKnee_flg]  "VTQD_ECPECASRKnee_flg"
  [VTQD_ECPECASRKnee_flg] -> DelayEnable5/1
  [VBCM_FDCBCMFDOpenSVCmd_flg] -> Detect Decrease6/1
  [VBCM_FDCBCMFDCloseSVCmd_flg] -> NOT1/1
  VTQD_ActFRDoorOPSta_flg/1 -> [VTQD_ActFRDoorOPSta_flg]
  Detect Decrease6/1 -> AND9/1
  NOT1/1 -> AND9/2
  [VTQD_ActFRDoorOPSta_flg] -> AND9/3
  AND9/1 -> [VTQD_ComboKeyReset_flg]  "VTQD_ComboKeyReset_flg"
  Constant6/1 -> Equal13/2
  [VINP_TransReqGear_enum] -> Equal13/1
  Equal13/1 -> AND7/1
  Constant7/1 -> Equal14/2
  Equal14/1 -> AND7/2
  [VINP_TransReqGear_enum] -> Equal14/1
  AND7/1 -> SR_Latch1/1
  [VINP_TransReqGear_enum] -> Equal16/1
  Constant9/1 -> Equal16/2
  [VINP_TransReqGear_enum] -> Delay2/1
  Delay2/1 -> Equal15/1
  Constant8/1 -> Equal15/2
  SR_Latch1/1 -> AND10/1  "VTQD_N2DEnterKeyReady_flg"
  Equal15/1 -> AND10/2
  Equal16/1 -> AND10/3
  AND10/1 -> SR_Latch2/1
  Delay3/1 -> Equal17/1
  [VINP_TransReqGear_enum] -> Delay3/1
  Constant27/1 -> Equal18/2
  Equal17/1 -> AND11/2
  [VINP_TransReqGear_enum] -> Equal18/1
  Constant10/1 -> Equal17/2
  Equal18/1 -> AND11/3
  SR_Latch2/1 -> AND11/1  "VTQD_D2REnterKeyReady_flg"
  SR_Latch3/1 -> AND12/1  "VTQD_R2NEnterKeyReady_flg"
  AND11/1 -> SR_Latch3/1
  [VINP_TransReqGear_enum] -> Equal19/1
  Constant28/1 -> Equal19/2
  Equal19/1 -> AND12/2
  AND12/1 -> DelayEnable6/1
  [task_time_s] -> DelayEnable6/3
  Constant29/1 -> DelayEnable6/2
  [VTQD_ComboKeyEnter_flg] -> Delay/1
  Delay/1 -> Detect Increase1/1
  Detect Increase1/1 -> OR1/1
  NOT2/1 -> OR1/2
  OR1/1 -> SR_Latch3/2, SR_Latch2/2, SR_Latch1/2  "VTQD_EnterKeyRest_flg"
  Constant30/1 -> Street Fight Switch Off/2(VTQD_SWCCANCELStaShort_flg)  "VTQD_SWCCANCELStaShort_flg"
  Constant31/1 -> Street Fight Switch Off/4(SWCCANCELStaLong_flg)  "SWCCANCELStaLong_flg"
  Delay4/1 -> OR/1
  [VTQD_ComboKeyEnter_flg] -> Delay4/1
  [VTQD_ComboKeyEn_flg] -> NOT2/1
  [VTQD_ComboKeyEn_flg] -> AND7/3
  [VTQD_ComboKeyEn_flg] -> AND10/4
  [VTQD_ComboKeyEn_flg] -> AND11/4
  [VTQD_ComboKeyEn_flg] -> AND12/3
  [VTQD_ComboKeyEn_flg] -> AND9/4

== system tqd/TQD/Input_Convert/Input Signal Convert/Big Mike Combo V2 /Combo Key Detection/Function1 Alcohol Lock ==
  note: Street Fight Mode:
      | 3 = VINP_SWC2LScrollUpSta_flg
      | 3 = VINP_SWC2LScrollUpSta_flg
      | 4 = VINP_SWC2LScrollDownSta_flg
      | 4 = VINP_SWC2LScrollDownSta_flg
      | 1 = VINP_SWC2RegenDown_flg
      | 1 = VINP_SWC2RegenDown_flg
      | 2 = VINP_SWC2RegenUp_flg
      | 2 = VINP_SWC2RegenUp_flg
  task_time_s : Inport
  VTQD_ComboKeyEn_flg : Inport  Port=2
  VTQD_ComboKeyReset_flg : Inport  Port=3
  VTQD_ComboKey_enum : Inport  Port=4
  VTQD_ComboKeyEnter_flg : Inport  Port=5
  VTQD_ComboKeyOff_flg : Inport  Port=6
  AND : Logic  Inputs=9  AllPortsSameDT=off  OutDataTypeStr=boolean
  AND1 : Logic  AllPortsSameDT=off  OutDataTypeStr=boolean
  Constant : Constant  Value=ENUM_COMBOKEY_NONE
  Constant1 : Constant  Value=ENUM_COMBOKEY_NONE
  Constant2 : Constant  Value=FALSE
  Constant3 : Constant  Value=KTQD_ComboKeyDelay_s
  Delay : Delay  DelayLength=1  InitialCondition=boolean(0)
      settings: AttributesFormatString=%<InitialCondition>
  Delay1 : Delay  DelayLength=1  InitialCondition=boolean(0)
      settings: AttributesFormatString=%<InitialCondition>
  DelayEnable : hcu_lib/Basic_Blocks/DelayEnable
  Equal : RelationalOperator  Operator=~=  OutDataTypeStr=boolean  RndMeth=Simplest
  Key1 : Subsystem
      settings: RTWSystemCode=Nonreusable function
  Key2 : Subsystem
      settings: RTWSystemCode=Nonreusable function
  Key3 : Subsystem
      settings: RTWSystemCode=Nonreusable function
  Key4 : Subsystem
      settings: RTWSystemCode=Nonreusable function
  Key5 : Subsystem
      settings: RTWSystemCode=Nonreusable function
  Key6 : Subsystem
      settings: RTWSystemCode=Nonreusable function
  Key7 : Subsystem
      settings: RTWSystemCode=Nonreusable function
  Key8 : Subsystem
      settings: RTWSystemCode=Nonreusable function
  NOT : Logic  Operator=NOT  AllPortsSameDT=off  OutDataTypeStr=boolean
  Switch : Switch  Criteria=u2 ~= 0
      settings: AttributesFormatString=%<Criteria>
  Switch1 : Switch  Criteria=u2 ~= 0
      settings: AttributesFormatString=%<Criteria>
  Switch2 : Switch  Criteria=u2 ~= 0
      settings: AttributesFormatString=%<Criteria>
  VTQD_Function1Off_flg : Outport
  wires:
  Switch/1 -> [VTQD_Function1CMD_enum]  "VTQD_Function1CMD_enum"
  [task_time_s] -> DelayEnable/3
  Constant/1 -> Switch/3
  DelayEnable/1 -> Switch/2
  [VTQD_ComboKeyEn_flg] -> DelayEnable/1
  Constant3/1 -> DelayEnable/2
  [VTQD_ComboKey_enum] -> Switch/1
  [VTQD_Function1CMD_enum] -> Key1/1(VTQD_ComboKeyCMD_enum)
  [VTQD_ComboKeyEn_flg] -> Key1/2(VTQD_ComboKeyEn_flg)
  [VTQD_ComboKeyReset_flg] -> Key1/3(VTQD_ComboKeyReset_flg)
  [VTQD_Function1CMD_enum] -> Key2/1(VTQD_Function1CMD_enum)
  [VTQD_ComboKeyEn_flg] -> Key2/2(VTQD_ComboKeyEn_flg)
  [VTQD_ComboKeyReset_flg] -> Key2/3(VTQD_ComboKeyReset_flg)
  [VTQD_ComboKey1_enum] -> Key2/4(VTQD_ComboKey1_enum)
  Key1/1(VTQD_ComboKey1_enum) -> [VTQD_ComboKey1_enum]
  Key1/2(VTQD_Key1Pass_flg) -> [VTQD_Key1Pass_flg]
  [VTQD_Function1CMD_enum] -> Key3/1(VTQD_ComboKeyCMD_enum)
  [VTQD_ComboKeyEn_flg] -> Key3/2(VTQD_ComboKeyEn_flg)
  [VTQD_ComboKeyReset_flg] -> Key3/3(VTQD_ComboKeyReset_flg)
  [VTQD_ComboKey2_enum] -> Key3/4(VTQD_ComboKey2_enum)
  [VTQD_Function1CMD_enum] -> Key4/1(VTQD_ComboKeyCMD_enum)
  [VTQD_ComboKeyEn_flg] -> Key4/2(VTQD_ComboKeyEn_flg)
  [VTQD_ComboKeyReset_flg] -> Key4/3(VTQD_ComboKeyReset_flg)
  Key2/1(VTQD_ComboKey2_enum) -> [VTQD_ComboKey2_enum]
  Key2/2(VTQD_Key2Pass_flg) -> [VTQD_Key2Pass_flg]
  [VTQD_ComboKey3_enum] -> Key4/4(VTQD_ComboKey3_enum)
  Key3/1(VTQD_ComboKey3_enum) -> [VTQD_ComboKey3_enum]
  Key3/2(VTQD_Key3Pass_flg) -> [VTQD_Key3Pass_flg]
  Key4/1(VTQD_ComboKey4_enum) -> [VTQD_ComboKey4_enum]
  Key4/2(VTQD_Key4Pass_flg) -> [VTQD_Key4Pass_flg]
  [VTQD_ComboKeyReset_flg] -> Key5/3(VTQD_ComboKeyReset_flg)
  [VTQD_ComboKeyEn_flg] -> Key5/2(VTQD_ComboKeyEn_flg)
  [VTQD_Function1CMD_enum] -> Key5/1(VTQD_ComboKeyCMD_enum)
  [VTQD_ComboKey4_enum] -> Key5/4(VTQD_ComboKey4_enum)
  Key5/2(VTQD_Key5Pass_flg) -> [VTQD_Key5Pass_flg]
  Key5/1(VTQD_ComboKey5_enum) -> [VTQD_ComboKey5_enum]
  Key7/2(VTQD_Key7Pass_flg) -> [VTQD_Key7Pass_flg]
  Key8/1(VTQD_ComboKey8_enum) -> [VTQD_ComboKey8_enum]
  Key8/2(VTQD_Key8Pass_flg) -> [VTQD_Key8Pass_flg]
  [VTQD_Function1CMD_enum] -> Key6/1(VTQD_ComboKeyCMD_enum)
  [VTQD_ComboKeyEn_flg] -> Key6/2(VTQD_ComboKeyEn_flg)
  [VTQD_ComboKeyReset_flg] -> Key6/3(VTQD_ComboKeyReset_flg)
  [VTQD_ComboKey5_enum] -> Key6/4(VTQD_ComboKey5_enum)
  [VTQD_Function1CMD_enum] -> Key7/1(VTQD_ComboKeyCMD_enum)
  [VTQD_ComboKeyEn_flg] -> Key7/2(VTQD_ComboKeyEn_flg)
  [VTQD_ComboKeyReset_flg] -> Key7/3(VTQD_ComboKeyReset_flg)
  [VTQD_ComboKey6_enum] -> Key7/4(VTQD_ComboKey6_enum)
  [VTQD_Function1CMD_enum] -> Key8/1(VTQD_ComboKeyCMD_enum)
  [VTQD_ComboKeyEn_flg] -> Key8/2(VTQD_ComboKeyEn_flg)
  [VTQD_ComboKeyReset_flg] -> Key8/3(VTQD_ComboKeyReset_flg)
  [VTQD_ComboKey7_enum] -> Key8/4(VTQD_ComboKey7_enum)
  Constant1/1 -> Equal/2
  Equal/1 -> AND/1
  [VTQD_Key1Pass_flg] -> AND/2
  [VTQD_Key8Pass_flg] -> AND/9
  [VTQD_Key7Pass_flg] -> AND/8
  [VTQD_Key6Pass_flg] -> AND/7
  [VTQD_Key5Pass_flg] -> AND/6
  [VTQD_Key4Pass_flg] -> AND/5
  [VTQD_Key3Pass_flg] -> AND/4
  [VTQD_Key2Pass_flg] -> AND/3
  AND/1 -> Switch1/1  "VTQD_Function1OffPass_flg"
  Switch1/1 -> Switch2/3
  [VTQD_ComboKeyOff_flg] -> Switch2/2
  Constant2/1 -> Switch2/1
  Switch2/1 -> [VTQD_Function1Off_flg], Delay/1  "VTQD_Function1Off_flg"
  Delay/1 -> Switch1/3
  task_time_s/1 -> [task_time_s]
  VTQD_ComboKeyEn_flg/1 -> [VTQD_ComboKeyEn_flg]
  VTQD_ComboKeyReset_flg/1 -> [VTQD_ComboKeyReset_flg]
  VTQD_ComboKey_enum/1 -> [VTQD_ComboKey_enum]
  VTQD_ComboKeyEnter_flg/1 -> [VTQD_ComboKeyEnter_flg]
  VTQD_ComboKeyOff_flg/1 -> [VTQD_ComboKeyOff_flg]
  [VTQD_Function1Off_flg] -> VTQD_Function1Off_flg/1
  Key6/1(VTQD_ComboKey6_enum) -> [VTQD_ComboKey6_enum]
  Key6/2(VTQD_Key6Pass_flg) -> [VTQD_Key6Pass_flg]
  Key7/1(VTQD_ComboKey7_enum) -> [VTQD_ComboKey7_enum]
  [VTQD_ComboKey8_enum] -> Equal/1
  AND1/1 -> Switch1/2
  [VTQD_ComboKeyEnter_flg] -> AND1/1
  NOT/1 -> AND1/2
  Delay1/1 -> NOT/1
  [VTQD_Function1Off_flg] -> Delay1/1

== system tqd/TQD/Input_Convert/Input Signal Convert/Big Mike Combo V2 /Combo Key Detection/Function2  ==
  note: Engineering Mode:
      | 5 = VINP_SWC2RScrollUpSta_flg
      | 5 = VINP_SWC2RScrollUpSta_flg
      | 6 = VINP_SWC2RScrollDownSta_flg
      | 6 = VINP_SWC2RScrollDownSta_flg
      | 5 = VINP_SWC2RScrollUpSta_flg
      | 6 = VINP_SWC2RScrollDownSta_flg
      | 5 = VINP_SWC2RScrollUpSta_flg
      | 6 = VINP_SWC2RScrollDownSta_flg
  task_time_s : Inport
  VTQD_ComboKeyEn_flg : Inport  Port=2
  VTQD_ComboKeyReset_flg : Inport  Port=3
  VTQD_ComboKey_enum : Inport  Port=4
  VTQD_ComboKeyEnter_flg : Inport  Port=5
  VTQD_ComboKeyOff_flg : Inport  Port=6
  AND : Logic  Inputs=9  AllPortsSameDT=off  OutDataTypeStr=boolean
  AND1 : Logic  AllPortsSameDT=off  OutDataTypeStr=boolean
  Constant : Constant  Value=ENUM_COMBOKEY_NONE
  Constant1 : Constant  Value=ENUM_COMBOKEY_NONE
  Constant2 : Constant  Value=FALSE
  Constant3 : Constant  Value=KTQD_ComboKeyDelay_s
  Delay : Delay  DelayLength=1  InitialCondition=boolean(0)
      settings: AttributesFormatString=%<InitialCondition>
  Delay1 : Delay  DelayLength=1  InitialCondition=boolean(0)
      settings: AttributesFormatString=%<InitialCondition>
  DelayEnable : hcu_lib/Basic_Blocks/DelayEnable
  Equal : RelationalOperator  Operator=~=  OutDataTypeStr=boolean  RndMeth=Simplest
  Key1 : Subsystem
      settings: RTWSystemCode=Nonreusable function
  Key2 : Subsystem
      settings: RTWSystemCode=Nonreusable function
  Key3 : Subsystem
      settings: RTWSystemCode=Nonreusable function
  Key4 : Subsystem
      settings: RTWSystemCode=Nonreusable function
  Key5 : Subsystem
      settings: RTWSystemCode=Nonreusable function
  Key6 : Subsystem
      settings: RTWSystemCode=Nonreusable function
  Key7 : Subsystem
      settings: RTWSystemCode=Nonreusable function
  Key8 : Subsystem
      settings: RTWSystemCode=Nonreusable function
  NOT : Logic  Operator=NOT  AllPortsSameDT=off  OutDataTypeStr=boolean
  Switch : Switch  Criteria=u2 ~= 0
      settings: AttributesFormatString=%<Criteria>
  Switch1 : Switch  Criteria=u2 ~= 0
      settings: AttributesFormatString=%<Criteria>
  Switch2 : Switch  Criteria=u2 ~= 0
      settings: AttributesFormatString=%<Criteria>
  VTQD_Function2Off_flg : Outport
  wires:
  [VTQD_ComboKey8_enum] -> Equal/1
  Key7/1(VTQD_ComboKey7_enum) -> [VTQD_ComboKey7_enum]
  Key6/2(VTQD_Key6Pass_flg) -> [VTQD_Key6Pass_flg]
  Key6/1(VTQD_ComboKey6_enum) -> [VTQD_ComboKey6_enum]
  VTQD_ComboKeyOff_flg/1 -> [VTQD_ComboKeyOff_flg]
  VTQD_ComboKeyEnter_flg/1 -> [VTQD_ComboKeyEnter_flg]
  VTQD_ComboKey_enum/1 -> [VTQD_ComboKey_enum]
  VTQD_ComboKeyReset_flg/1 -> [VTQD_ComboKeyReset_flg]
  VTQD_ComboKeyEn_flg/1 -> [VTQD_ComboKeyEn_flg]
  task_time_s/1 -> [task_time_s]
  Delay/1 -> Switch1/3
  Switch2/1 -> [VTQD_Function2Off_flg], Delay/1  "VTQD_Function2Off_flg"
  Constant2/1 -> Switch2/1
  [VTQD_ComboKeyOff_flg] -> Switch2/2
  Switch1/1 -> Switch2/3
  AND/1 -> Switch1/1  "VTQD_Function2OffPass_flg"
  [VTQD_Key2Pass_flg] -> AND/3
  [VTQD_Key3Pass_flg] -> AND/4
  [VTQD_Key4Pass_flg] -> AND/5
  [VTQD_Key5Pass_flg] -> AND/6
  [VTQD_Key6Pass_flg] -> AND/7
  [VTQD_Key7Pass_flg] -> AND/8
  [VTQD_Key8Pass_flg] -> AND/9
  [VTQD_Key1Pass_flg] -> AND/2
  Equal/1 -> AND/1
  Constant1/1 -> Equal/2
  [VTQD_ComboKey7_enum] -> Key8/4(VTQD_ComboKey7_enum)
  [VTQD_ComboKeyReset_flg] -> Key8/3(VTQD_ComboKeyReset_flg)
  [VTQD_ComboKeyEn_flg] -> Key8/2(VTQD_ComboKeyEn_flg)
  [VTQD_Function2CMD_enum] -> Key8/1(VTQD_ComboKeyCMD_enum)
  [VTQD_ComboKey6_enum] -> Key7/4(VTQD_ComboKey6_enum)
  [VTQD_ComboKeyReset_flg] -> Key7/3(VTQD_ComboKeyReset_flg)
  [VTQD_ComboKeyEn_flg] -> Key7/2(VTQD_ComboKeyEn_flg)
  [VTQD_Function2CMD_enum] -> Key7/1(VTQD_ComboKeyCMD_enum)
  [VTQD_ComboKey5_enum] -> Key6/4(VTQD_ComboKey5_enum)
  [VTQD_ComboKeyReset_flg] -> Key6/3(VTQD_ComboKeyReset_flg)
  [VTQD_ComboKeyEn_flg] -> Key6/2(VTQD_ComboKeyEn_flg)
  [VTQD_Function2CMD_enum] -> Key6/1(VTQD_ComboKeyCMD_enum)
  Key8/2(VTQD_Key8Pass_flg) -> [VTQD_Key8Pass_flg]
  Key8/1(VTQD_ComboKey8_enum) -> [VTQD_ComboKey8_enum]
  Key7/2(VTQD_Key7Pass_flg) -> [VTQD_Key7Pass_flg]
  Key5/1(VTQD_ComboKey5_enum) -> [VTQD_ComboKey5_enum]
  Key5/2(VTQD_Key5Pass_flg) -> [VTQD_Key5Pass_flg]
  [VTQD_ComboKey4_enum] -> Key5/4(VTQD_ComboKey4_enum)
  [VTQD_Function2CMD_enum] -> Key5/1(VTQD_ComboKeyCMD_enum)
  [VTQD_ComboKeyEn_flg] -> Key5/2(VTQD_ComboKeyEn_flg)
  [VTQD_ComboKeyReset_flg] -> Key5/3(VTQD_ComboKeyReset_flg)
  Key4/2(VTQD_Key4Pass_flg) -> [VTQD_Key4Pass_flg]
  Key4/1(VTQD_ComboKey4_enum) -> [VTQD_ComboKey4_enum]
  Key3/2(VTQD_Key3Pass_flg) -> [VTQD_Key3Pass_flg]
  Key3/1(VTQD_ComboKey3_enum) -> [VTQD_ComboKey3_enum]
  [VTQD_ComboKey3_enum] -> Key4/4(VTQD_ComboKey3_enum)
  Key2/2(VTQD_Key2Pass_flg) -> [VTQD_Key2Pass_flg]
  Key2/1(VTQD_ComboKey2_enum) -> [VTQD_ComboKey2_enum]
  [VTQD_ComboKeyReset_flg] -> Key4/3(VTQD_ComboKeyReset_flg)
  [VTQD_ComboKeyEn_flg] -> Key4/2(VTQD_ComboKeyEn_flg)
  [VTQD_Function2CMD_enum] -> Key4/1(VTQD_ComboKeyCMD_enum)
  [VTQD_ComboKey2_enum] -> Key3/4(VTQD_ComboKey2_enum)
  [VTQD_ComboKeyReset_flg] -> Key3/3(VTQD_ComboKeyReset_flg)
  [VTQD_ComboKeyEn_flg] -> Key3/2(VTQD_ComboKeyEn_flg)
  [VTQD_Function2CMD_enum] -> Key3/1(VTQD_ComboKeyCMD_enum)
  Key1/2(VTQD_Key1Pass_flg) -> [VTQD_Key1Pass_flg]
  Key1/1(VTQD_ComboKey1_enum) -> [VTQD_ComboKey1_enum]
  [VTQD_ComboKey1_enum] -> Key2/4(VTQD_ComboKey1_enum)
  [VTQD_ComboKeyReset_flg] -> Key2/3(VTQD_ComboKeyReset_flg)
  [VTQD_ComboKeyEn_flg] -> Key2/2(VTQD_ComboKeyEn_flg)
  [VTQD_Function2CMD_enum] -> Key2/1(VTQD_ComboKeyCMD_enum)
  [VTQD_ComboKeyReset_flg] -> Key1/3(VTQD_ComboKeyReset_flg)
  [VTQD_ComboKeyEn_flg] -> Key1/2(VTQD_ComboKeyEn_flg)
  [VTQD_Function2CMD_enum] -> Key1/1(VTQD_ComboKeyCMD_enum)
  [VTQD_ComboKey_enum] -> Switch/1
  Constant3/1 -> DelayEnable/2
  [VTQD_ComboKeyEn_flg] -> DelayEnable/1
  DelayEnable/1 -> Switch/2
  Constant/1 -> Switch/3
  [task_time_s] -> DelayEnable/3
  Switch/1 -> [VTQD_Function2CMD_enum]  "VTQD_Function2CMD_enum"
  [VTQD_Function2Off_flg] -> VTQD_Function2Off_flg/1
  [VTQD_ComboKeyEnter_flg] -> AND1/1
  AND1/1 -> Switch1/2
  [VTQD_Function2Off_flg] -> Delay1/1
  Delay1/1 -> NOT/1
  NOT/1 -> AND1/2
